simulink library "CgCp_ul"  (R2020a)
settings: Solver=VariableStepAuto  StartTime=0.0  StopTime=10.0  RelTol=1e-3
undefined symbols (not defined in the file): Veh
settings Model: Creator=bunce  LastModifiedBy=bunce

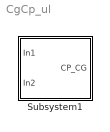
== system CgCp_ul ==
  Subsystem1 : Subsystem

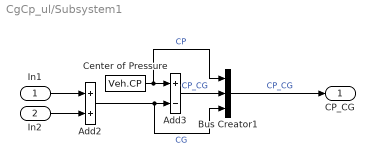
== system CgCp_ul/Subsystem1 ==
  In1 : Inport
  In2 : Inport  Port=2
  Add2 : Sum
  Add3 : Sum  Inputs=+-
  Bus Creator1 : BusCreator  Inputs=3
  Center of Pressure : Constant  Value=Veh.CP
  CP_CG : Outport
  wires:
  Center of Pressure/1 -> Bus Creator1/1, Add3/1  "CP"
  Add3/1 -> Bus Creator1/2  "CP_CG"
  Bus Creator1/1 -> CP_CG/1  "CP_CG"
  Add2/1 -> Bus Creator1/3, Add3/2  "CG"
  In1/1 -> Add2/1
  In2/1 -> Add2/2
